simulink model "System"  (R2024a)
settings: Solver=ode45  StartTime=0.0  StopTime=5  RelTol=1e-3
InitFcn:
  | load('parameters.mat')
values from neighbouring files (symbols this model uses):
  Q_KF = diag([0 1e-1 1 1 0])    [Main.m]
  R_KF = diag(1e-8)    [Main.m]
undefined symbols (not defined in the file or in its folder): alpha0
settings Model: Creator=Bocchio  LastModifiedBy=Bocchio

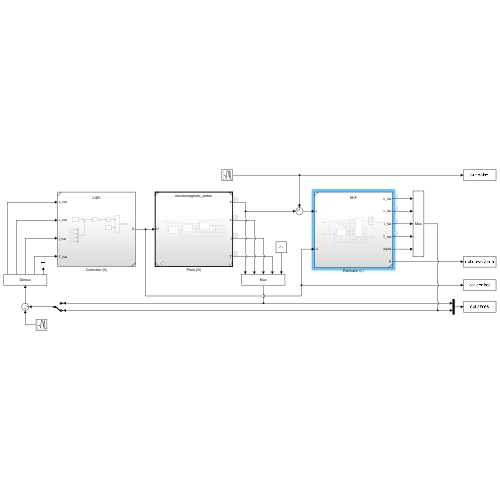
[thumbnail: Simulink's stored preview of the top-level diagram]
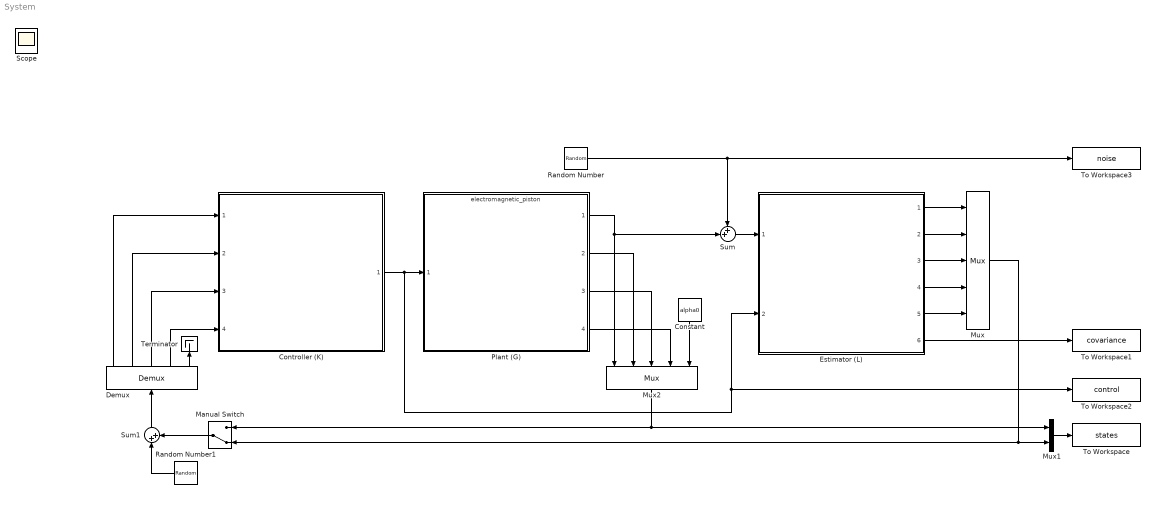
== system System ==
  Constant : Constant  Value=alpha0
  Controller (K) : Subsystem  ReferencedSubsystem=LQR
  Demux : Demux  Outputs=5
      settings: DisplayOption=none
  Estimator (L) : Subsystem  ReferencedSubsystem=EKF
  Manual Switch : ManualSwitch  CurrentSetting=0
  Mux : Mux  Inputs=5
  Mux1 : Mux  Inputs=2
  Mux2 : Mux  Inputs=5
  Plant (G) : ModelReference  ModelNameDialog=electromagnetic_piston.slx  SimulationMode=Normal  ModelReferenceVersion=1.20
  Random Number : RandomNumber  Variance=diag(R_KF)  SampleTime=0.002
  Random Number1 : RandomNumber  Variance=diag(Q_KF)  Seed=[0 10 20 30 40]  SampleTime=0.002
  Sum : Sum  Inputs=++|
  Sum1 : Sum  Inputs=|++
  Terminator : Terminator
  To Workspace : ToWorkspace  VariableName=states  SaveFormat=Timeseries  SampleTime=-1
  To Workspace1 : ToWorkspace  VariableName=covariance  SaveFormat=Timeseries  SampleTime=-1
  To Workspace2 : ToWorkspace  VariableName=control  SaveFormat=Timeseries  SampleTime=-1
  To Workspace3 : ToWorkspace  VariableName=noise  SaveFormat=Timeseries  SampleTime=-1
  Scope : Scope
  wires:
  Estimator (L)/1 -> Mux/1
  Estimator (L)/2 -> Mux/2
  Estimator (L)/3 -> Mux/3
  Mux/1 -> Mux1/2, Manual Switch/2
  Demux/1 -> Controller (K)/1
  Demux/2 -> Controller (K)/2
  Demux/3 -> Controller (K)/3
  Demux/4 -> Controller (K)/4
  Estimator (L)/4 -> Mux/4
  Mux1/1 -> To Workspace/1
  Plant (G)/2 -> Mux2/2
  Plant (G)/3 -> Mux2/3
  Plant (G)/4 -> Mux2/4
  Mux2/1 -> Manual Switch/1, Mux1/1
  Estimator (L)/5 -> Mux/5
  Estimator (L)/6 -> To Workspace1/1
  Manual Switch/1 -> Sum1/2
  Controller (K)/1 -> Estimator (L)/2, To Workspace2/1, Plant (G)/1
  Constant/1 -> Mux2/5
  Random Number/1 -> To Workspace3/1, Sum/1
  Sum1/1 -> Demux/1
  Random Number1/1 -> Sum1/1
  Demux/5 -> Terminator/1
  Sum/1 -> Estimator (L)/1
  Plant (G)/1 -> Mux2/1, Sum/2
